simulink model "EISGov_SelectParameter"  (R2016b)
settings: configuration reference "CodeGenConfigSet" (kept outside this file)
values from neighbouring files (symbols this model uses):
  EISGov_SetPLoRmpSlopeNeg_C = Calibration.Parameter    [init_EISGov_SelectParameter.m]    (also in init_EISGov_SelectParameter_SIL.m = Simulink.Parameter)
  EISGov_SetPLoRmpSlopePos_C = Calibration.Parameter    [init_EISGov_SelectParameter.m]    (also in init_EISGov_SelectParameter_SIL.m = Simulink.Parameter)
  EISGov_stPrio_CA = Calibration.Parameter    [init_EISGov_SelectParameter.m]    (also in init_EISGov_SelectParameter_SIL.m = Simulink.Parameter)
undefined symbols (not defined in the file or in its folder): EISGov_num_conv, EISGov_SelectParameter_DT, Switch_conv
libraries: simulink x20, CXLib x3
(part 2 of 2)

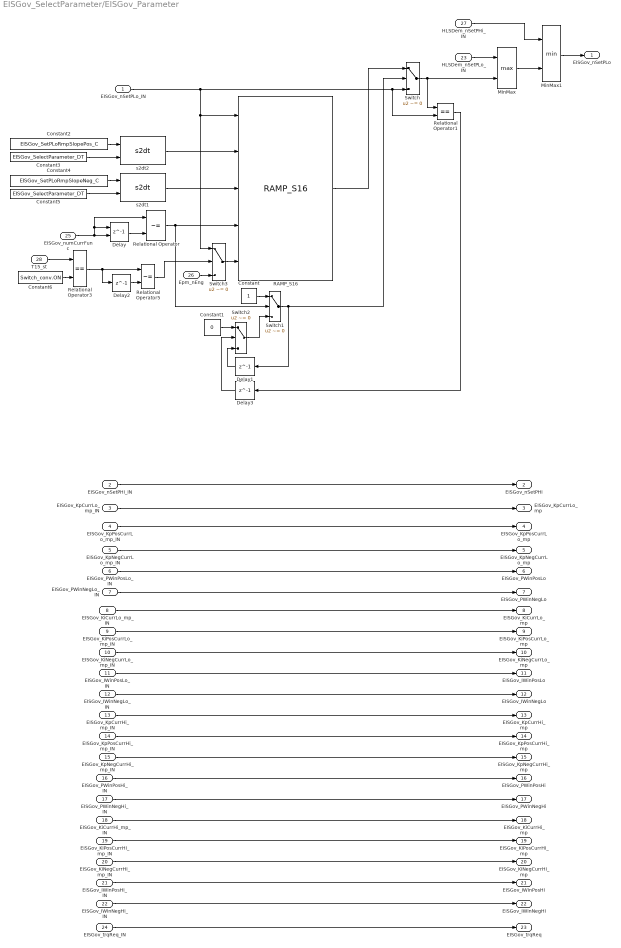
== system EISGov_SelectParameter/EISGov_Parameter ==
  EISGov_nSetPLo_IN : Inport
  EISGov_nSetPHi_IN : Inport  Port=2
  EISGov_KpCurrLo_mp_IN : Inport  Port=3
  EISGov_KpPosCurrLo_mp_IN : Inport  Port=4
  EISGov_KpNegCurrLo_mp_IN : Inport  Port=5
  EISGov_PWinPosLo_IN : Inport  Port=6
  EISGov_PWinNegLo_IN : Inport  Port=7
  EISGov_KiCurrLo_mp_IN : Inport  Port=8
  EISGov_KiPosCurrLo_mp_IN : Inport  Port=9
  EISGov_KiNegCurrLo_mp_IN : Inport  Port=10
  EISGov_IWinPosLo_IN : Inport  Port=11
  EISGov_IWinNegLo_IN : Inport  Port=12
  EISGov_KpCurrHi_mp_IN : Inport  Port=13
  EISGov_KpPosCurrHi_mp_IN : Inport  Port=14
  EISGov_KpNegCurrHi_mp_IN : Inport  Port=15
  EISGov_PWinPosHi_IN : Inport  Port=16
  EISGov_PWinNegHi_IN : Inport  Port=17
  EISGov_KiCurrHi_mp_IN : Inport  Port=18
  EISGov_KiPosCurrHi_mp_IN : Inport  Port=19
  EISGov_KiNegCurrHi_mp_IN : Inport  Port=20
  EISGov_IWinPosHi_IN : Inport  Port=21
  EISGov_IWinNegHi_IN : Inport  Port=22
  HLSDem_nSetPLo_IN : Inport  Port=23
  EISGov_trqReq_IN : Inport  Port=24
  EISGov_numCurrFunc : Inport  Port=25
  Epm_nEng : Inport  Tag=rpm  Description=Engine speed  Port=26  OutMin=0  OutMax=6000  OutDataTypeStr=EngSpeed_rpm
  HLSDem_nSetPHi_IN : Inport  Port=27
  T15_st : Inport  Port=28
  Constant : Constant  OutDataTypeStr=boolean
  Constant1 : Constant  Value=0  OutDataTypeStr=Inherit: Inherit via back propagation
  Constant2 : Constant  Value=EISGov_SetPLoRmpSlopePos_C
  Constant3 : Constant  Value=EISGov_SelectParameter_DT
  Constant4 : Constant  Value=EISGov_SetPLoRmpSlopeNeg_C
  Constant5 : Constant  Value=EISGov_SelectParameter_DT
  Constant6 : Constant  Value=Switch_conv.ON
  Delay : Delay  DelayLength=1  InitialConditionSource=Input port  InitialCondition=0
      settings: InputPortMap=u0,p4
  Delay1 : Delay  DelayLength=1  InitialCondition=0
  Delay2 : Delay  DelayLength=1  InitialCondition=0
  Delay3 : Delay  DelayLength=1  InitialCondition=0
  MinMax : MinMax  Function=max  Inputs=2
  MinMax1 : MinMax  Inputs=2
  RAMP_S16 : CXLib/RAMP_S16
  Relational Operator : RelationalOperator  Operator=~=  OutDataTypeStr=boolean  RndMeth=Simplest
  Relational Operator1 : RelationalOperator  Operator===  OutDataTypeStr=boolean  RndMeth=Simplest
  Relational Operator3 : RelationalOperator  Operator===  OutDataTypeStr=boolean  RndMeth=Simplest
  Relational Operator5 : RelationalOperator  Operator=~=  OutDataTypeStr=boolean  RndMeth=Simplest
  Switch{,1..3} (4 alike) : Switch  Criteria=u2 ~= 0
  s2dt1 : CXLib/s2dt
  s2dt2 : CXLib/s2dt
  EISGov_nSetPLo : Outport
  EISGov_nSetPHi : Outport  Port=2
  EISGov_KpCurrLo_mp : Outport  Port=3
  EISGov_KpPosCurrLo_mp : Outport  Port=4
  EISGov_KpNegCurrLo_mp : Outport  Port=5
  EISGov_PWinPosLo : Outport  Port=6
  EISGov_PWinNegLo : Outport  Port=7
  EISGov_KiCurrLo_mp : Outport  Port=8
  EISGov_KiPosCurrLo_mp : Outport  Port=9
  EISGov_KiNegCurrLo_mp : Outport  Port=10
  EISGov_IWinPosLo : Outport  Port=11
  EISGov_IWinNegLo : Outport  Port=12
  EISGov_KpCurrHi_mp : Outport  Port=13
  EISGov_KpPosCurrHi_mp : Outport  Port=14
  EISGov_KpNegCurrHi_mp : Outport  Port=15
  EISGov_PWinPosHi : Outport  Port=16
  EISGov_PWinNegHi : Outport  Port=17
  EISGov_KiCurrHi_mp : Outport  Port=18
  EISGov_KiPosCurrHi_mp : Outport  Port=19
  EISGov_KiNegCurrHi_mp : Outport  Port=20
  EISGov_IWinPosHi : Outport  Port=21
  EISGov_IWinNegHi : Outport  Port=22
  EISGov_trqReq : Outport  Port=23
  wires:
  EISGov_KpCurrLo_mp_IN/1 -> EISGov_KpCurrLo_mp/1
  EISGov_KpPosCurrLo_mp_IN/1 -> EISGov_KpPosCurrLo_mp/1
  EISGov_nSetPHi_IN/1 -> EISGov_nSetPHi/1
  EISGov_KiCurrLo_mp_IN/1 -> EISGov_KiCurrLo_mp/1
  EISGov_KiPosCurrHi_mp_IN/1 -> EISGov_KiPosCurrHi_mp/1
  EISGov_IWinNegLo_IN/1 -> EISGov_IWinNegLo/1
  EISGov_KpNegCurrHi_mp_IN/1 -> EISGov_KpNegCurrHi_mp/1
  EISGov_KiNegCurrHi_mp_IN/1 -> EISGov_KiNegCurrHi_mp/1
  EISGov_IWinPosLo_IN/1 -> EISGov_IWinPosLo/1
  EISGov_PWinPosHi_IN/1 -> EISGov_PWinPosHi/1
  EISGov_IWinNegHi_IN/1 -> EISGov_IWinNegHi/1
  EISGov_KiPosCurrLo_mp_IN/1 -> EISGov_KiPosCurrLo_mp/1
  EISGov_IWinPosHi_IN/1 -> EISGov_IWinPosHi/1
  EISGov_PWinNegHi_IN/1 -> EISGov_PWinNegHi/1
  EISGov_PWinPosLo_IN/1 -> EISGov_PWinPosLo/1
  EISGov_KpNegCurrLo_mp_IN/1 -> EISGov_KpNegCurrLo_mp/1
  EISGov_PWinNegLo_IN/1 -> EISGov_PWinNegLo/1
  EISGov_KpCurrHi_mp_IN/1 -> EISGov_KpCurrHi_mp/1
  EISGov_KiNegCurrLo_mp_IN/1 -> EISGov_KiNegCurrLo_mp/1
  EISGov_KpPosCurrHi_mp_IN/1 -> EISGov_KpPosCurrHi_mp/1
  EISGov_KiCurrHi_mp_IN/1 -> EISGov_KiCurrHi_mp/1
  HLSDem_nSetPLo_IN/1 -> MinMax/1
  EISGov_trqReq_IN/1 -> EISGov_trqReq/1
  EISGov_numCurrFunc/1 -> Relational Operator/1, Delay/1, Delay/2
  Delay/1 -> Relational Operator/2
  Constant3/1 -> s2dt2/2
  Constant2/1 -> s2dt2/1
  s2dt2/1 -> RAMP_S16/2
  Constant5/1 -> s2dt1/2
  Constant4/1 -> s2dt1/1
  s2dt1/1 -> RAMP_S16/3
  EISGov_nSetPLo_IN/1 -> Relational Operator1/2, Switch/3, RAMP_S16/1, Switch3/1
  Relational Operator/1 -> Switch1/2, RAMP_S16/4
  MinMax1/1 -> EISGov_nSetPLo/1
  MinMax/1 -> MinMax1/2
  HLSDem_nSetPHi_IN/1 -> MinMax1/1
  Switch/1 -> MinMax/2, Relational Operator1/1
  Switch2/1 -> Switch1/3
  Switch1/1 -> Switch/2, Delay1/1
  Constant/1 -> Switch1/1
  Constant1/1 -> Switch2/1
  Delay1/1 -> Switch2/3
  RAMP_S16/1 -> Switch/1
  Constant6/1 -> Relational Operator3/2
  Delay2/1 -> Relational Operator5/2
  Relational Operator3/1 -> Delay2/1, Relational Operator5/1
  T15_st/1 -> Relational Operator3/1
  Epm_nEng/1 -> Switch3/3
  Switch3/1 -> RAMP_S16/5
  Relational Operator5/1 -> Switch3/2
  Delay3/1 -> Switch2/2
  Relational Operator1/1 -> Delay3/1

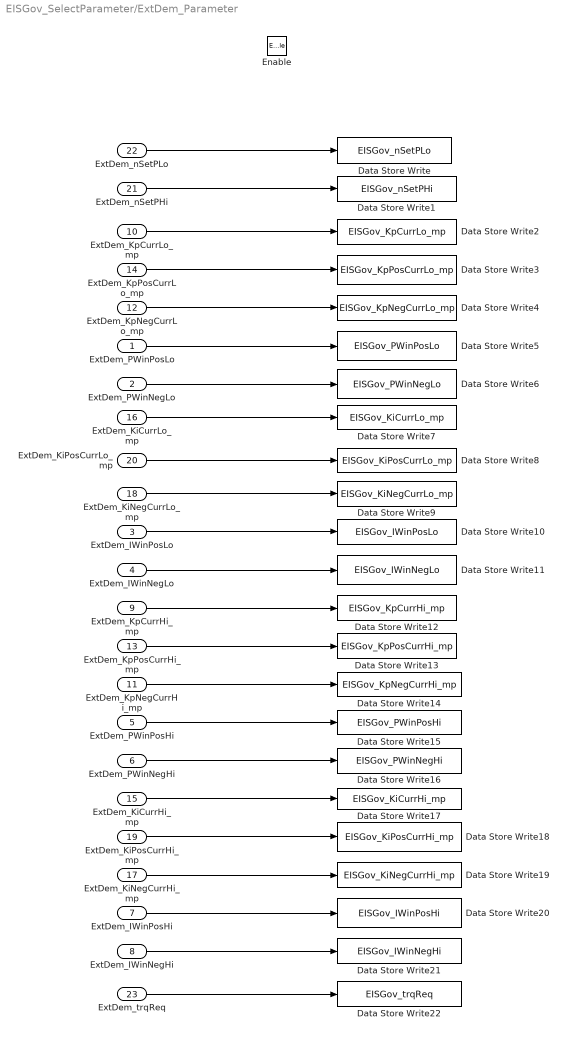
== system EISGov_SelectParameter/ExtDem_Parameter ==
  ExtDem_PWinPosLo : Inport  Tag=rpm  Description=P component Positive window for parameterset lower PI- path  OutMin=-6000  OutMax=6000  OutDataTypeStr=EngSpeed_rpm
  ExtDem_PWinNegLo : Inport  Tag=rpm  Description=P component negative window for parameterset lower PI- path  Port=2  OutMin=-6000  OutMax=6000  OutDataTypeStr=EngSpeed_rpm
  ExtDem_IWinPosLo : Inport  Tag=rpm  Description=I component Positive window for parameterset lower PI- path  Port=3  OutMin=-6000  OutMax=6000  OutDataTypeStr=EngSpeed_rpm
  ExtDem_IWinNegLo : Inport  Tag=rpm  Description=I component negative window for parameterset lower PI- path  Port=4  OutMin=-6000  OutMax=6000  OutDataTypeStr=EngSpeed_rpm
  ExtDem_PWinPosHi : Inport  Tag=rpm  Description=P component Positive window for parameterset upper PI- path  Port=5  OutMin=-6000  OutMax=6000  OutDataTypeStr=EngSpeed_rpm
  ExtDem_PWinNegHi : Inport  Tag=rpm  Description=P component negative window for parameterset upper PI- path  Port=6  OutMin=-6000  OutMax=6000  OutDataTypeStr=EngSpeed_rpm
  ExtDem_IWinPosHi : Inport  Tag=rpm  Description=I component Positive window for parameterset upper PI- path  Port=7  OutMin=-6000  OutMax=6000  OutDataTypeStr=EngSpeed_rpm
  ExtDem_IWinNegHi : Inport  Tag=rpm  Description=I component negative window for parameterset upper PI- path  Port=8  OutMin=-6000  OutMax=6000  OutDataTypeStr=EngSpeed_rpm
  ExtDem_KpCurrHi_mp : Inport  Port=9
  ExtDem_KpCurrLo_mp : Inport  Port=10
  ExtDem_KpNegCurrHi_mp : Inport  Port=11
  ExtDem_KpNegCurrLo_mp : Inport  Port=12
  ExtDem_KpPosCurrHi_mp : Inport  Port=13
  ExtDem_KpPosCurrLo_mp : Inport  Port=14
  ExtDem_KiCurrHi_mp : Inport  Port=15
  ExtDem_KiCurrLo_mp : Inport  Port=16
  ExtDem_KiNegCurrHi_mp : Inport  Port=17
  ExtDem_KiNegCurrLo_mp : Inport  Port=18
  ExtDem_KiPosCurrHi_mp : Inport  Port=19
  ExtDem_KiPosCurrLo_mp : Inport  Port=20
  ExtDem_nSetPHi : Inport  Port=21
  ExtDem_nSetPLo : Inport  Port=22
  ExtDem_trqReq : Inport  Port=23
  Enable : EnablePort
  Data Store Write : DataStoreWrite  DataStoreName=EISGov_nSetPLo
  Data Store Write1 : DataStoreWrite  DataStoreName=EISGov_nSetPHi
  Data Store Write10 : DataStoreWrite  DataStoreName=EISGov_IWinPosLo
  Data Store Write11 : DataStoreWrite  DataStoreName=EISGov_IWinNegLo
  Data Store Write12 : DataStoreWrite  DataStoreName=EISGov_KpCurrHi_mp
  Data Store Write13 : DataStoreWrite  DataStoreName=EISGov_KpPosCurrHi_mp
  Data Store Write14 : DataStoreWrite  DataStoreName=EISGov_KpNegCurrHi_mp
  Data Store Write15 : DataStoreWrite  DataStoreName=EISGov_PWinPosHi
  Data Store Write16 : DataStoreWrite  DataStoreName=EISGov_PWinNegHi
  Data Store Write17 : DataStoreWrite  DataStoreName=EISGov_KiCurrHi_mp
  Data Store Write18 : DataStoreWrite  DataStoreName=EISGov_KiPosCurrHi_mp
  Data Store Write19 : DataStoreWrite  DataStoreName=EISGov_KiNegCurrHi_mp
  Data Store Write2 : DataStoreWrite  DataStoreName=EISGov_KpCurrLo_mp
  Data Store Write20 : DataStoreWrite  DataStoreName=EISGov_IWinPosHi
  Data Store Write21 : DataStoreWrite  DataStoreName=EISGov_IWinNegHi
  Data Store Write22 : DataStoreWrite  DataStoreName=EISGov_trqReq
  Data Store Write3 : DataStoreWrite  DataStoreName=EISGov_KpPosCurrLo_mp
  Data Store Write4 : DataStoreWrite  DataStoreName=EISGov_KpNegCurrLo_mp
  Data Store Write5 : DataStoreWrite  DataStoreName=EISGov_PWinPosLo
  Data Store Write6 : DataStoreWrite  DataStoreName=EISGov_PWinNegLo
  Data Store Write7 : DataStoreWrite  DataStoreName=EISGov_KiCurrLo_mp
  Data Store Write8 : DataStoreWrite  DataStoreName=EISGov_KiPosCurrLo_mp
  Data Store Write9 : DataStoreWrite  DataStoreName=EISGov_KiNegCurrLo_mp
  wires:
  ExtDem_PWinPosLo/1 -> Data Store Write5/1
  ExtDem_PWinNegLo/1 -> Data Store Write6/1
  ExtDem_KiCurrLo_mp/1 -> Data Store Write7/1
  ExtDem_KiPosCurrLo_mp/1 -> Data Store Write8/1
  ExtDem_KiNegCurrLo_mp/1 -> Data Store Write9/1
  ExtDem_IWinPosLo/1 -> Data Store Write10/1
  ExtDem_IWinNegLo/1 -> Data Store Write11/1
  ExtDem_KpCurrHi_mp/1 -> Data Store Write12/1
  ExtDem_KpPosCurrHi_mp/1 -> Data Store Write13/1
  ExtDem_KpNegCurrHi_mp/1 -> Data Store Write14/1
  ExtDem_PWinPosHi/1 -> Data Store Write15/1
  ExtDem_PWinNegHi/1 -> Data Store Write16/1
  ExtDem_KiCurrHi_mp/1 -> Data Store Write17/1
  ExtDem_KiPosCurrHi_mp/1 -> Data Store Write18/1
  ExtDem_KiNegCurrHi_mp/1 -> Data Store Write19/1
  ExtDem_IWinPosHi/1 -> Data Store Write20/1
  ExtDem_IWinNegHi/1 -> Data Store Write21/1
  ExtDem_nSetPLo/1 -> Data Store Write/1
  ExtDem_nSetPHi/1 -> Data Store Write1/1
  ExtDem_KpCurrLo_mp/1 -> Data Store Write2/1
  ExtDem_KpPosCurrLo_mp/1 -> Data Store Write3/1
  ExtDem_KpNegCurrLo_mp/1 -> Data Store Write4/1
  ExtDem_trqReq/1 -> Data Store Write22/1

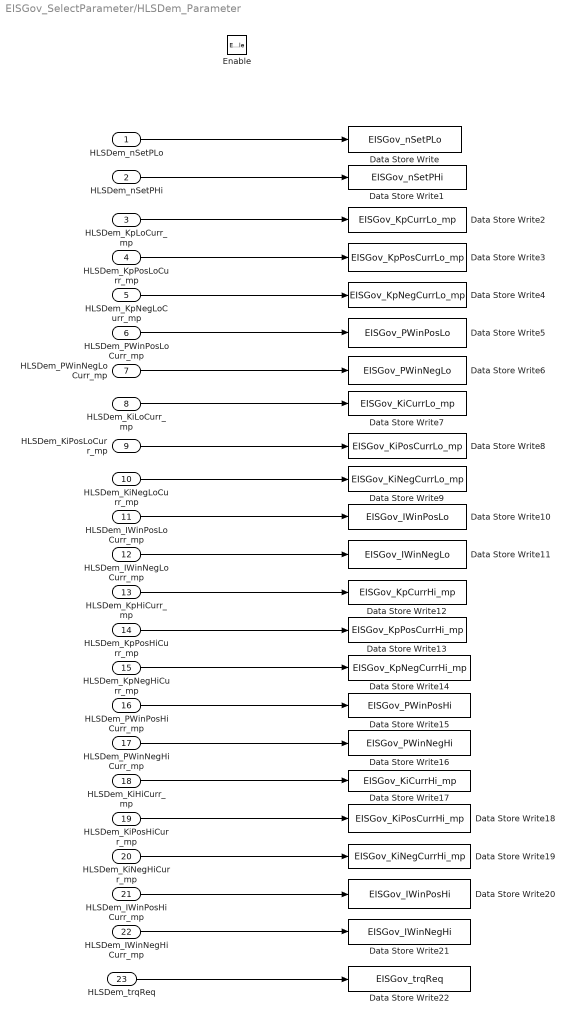
== system EISGov_SelectParameter/HLSDem_Parameter ==
  HLSDem_nSetPLo : Inport
  HLSDem_nSetPHi : Inport  Port=2
  HLSDem_KpLoCurr_mp : Inport  Port=3
  HLSDem_KpPosLoCurr_mp : Inport  Port=4
  HLSDem_KpNegLoCurr_mp : Inport  Port=5
  HLSDem_PWinPosLoCurr_mp : Inport  Port=6
  HLSDem_PWinNegLoCurr_mp : Inport  Port=7
  HLSDem_KiLoCurr_mp : Inport  Port=8
  HLSDem_KiPosLoCurr_mp : Inport  Port=9
  HLSDem_KiNegLoCurr_mp : Inport  Port=10
  HLSDem_IWinPosLoCurr_mp : Inport  Port=11
  HLSDem_IWinNegLoCurr_mp : Inport  Port=12
  HLSDem_KpHiCurr_mp : Inport  Port=13
  HLSDem_KpPosHiCurr_mp : Inport  Port=14
  HLSDem_KpNegHiCurr_mp : Inport  Port=15
  HLSDem_PWinPosHiCurr_mp : Inport  Port=16
  HLSDem_PWinNegHiCurr_mp : Inport  Port=17
  HLSDem_KiHiCurr_mp : Inport  Port=18
  HLSDem_KiPosHiCurr_mp : Inport  Port=19
  HLSDem_KiNegHiCurr_mp : Inport  Port=20
  HLSDem_IWinPosHiCurr_mp : Inport  Port=21
  HLSDem_IWinNegHiCurr_mp : Inport  Port=22
  HLSDem_trqReq : Inport  Port=23
  Enable : EnablePort
  Data Store Write : DataStoreWrite  DataStoreName=EISGov_nSetPLo
  Data Store Write1 : DataStoreWrite  DataStoreName=EISGov_nSetPHi
  Data Store Write10 : DataStoreWrite  DataStoreName=EISGov_IWinPosLo
  Data Store Write11 : DataStoreWrite  DataStoreName=EISGov_IWinNegLo
  Data Store Write12 : DataStoreWrite  DataStoreName=EISGov_KpCurrHi_mp
  Data Store Write13 : DataStoreWrite  DataStoreName=EISGov_KpPosCurrHi_mp
  Data Store Write14 : DataStoreWrite  DataStoreName=EISGov_KpNegCurrHi_mp
  Data Store Write15 : DataStoreWrite  DataStoreName=EISGov_PWinPosHi
  Data Store Write16 : DataStoreWrite  DataStoreName=EISGov_PWinNegHi
  Data Store Write17 : DataStoreWrite  DataStoreName=EISGov_KiCurrHi_mp
  Data Store Write18 : DataStoreWrite  DataStoreName=EISGov_KiPosCurrHi_mp
  Data Store Write19 : DataStoreWrite  DataStoreName=EISGov_KiNegCurrHi_mp
  Data Store Write2 : DataStoreWrite  DataStoreName=EISGov_KpCurrLo_mp
  Data Store Write20 : DataStoreWrite  DataStoreName=EISGov_IWinPosHi
  Data Store Write21 : DataStoreWrite  DataStoreName=EISGov_IWinNegHi
  Data Store Write22 : DataStoreWrite  DataStoreName=EISGov_trqReq
  Data Store Write3 : DataStoreWrite  DataStoreName=EISGov_KpPosCurrLo_mp
  Data Store Write4 : DataStoreWrite  DataStoreName=EISGov_KpNegCurrLo_mp
  Data Store Write5 : DataStoreWrite  DataStoreName=EISGov_PWinPosLo
  Data Store Write6 : DataStoreWrite  DataStoreName=EISGov_PWinNegLo
  Data Store Write7 : DataStoreWrite  DataStoreName=EISGov_KiCurrLo_mp
  Data Store Write8 : DataStoreWrite  DataStoreName=EISGov_KiPosCurrLo_mp
  Data Store Write9 : DataStoreWrite  DataStoreName=EISGov_KiNegCurrLo_mp
  wires:
  HLSDem_nSetPLo/1 -> Data Store Write/1
  HLSDem_nSetPHi/1 -> Data Store Write1/1
  HLSDem_KpLoCurr_mp/1 -> Data Store Write2/1
  HLSDem_KpPosLoCurr_mp/1 -> Data Store Write3/1
  HLSDem_KpNegLoCurr_mp/1 -> Data Store Write4/1
  HLSDem_PWinPosLoCurr_mp/1 -> Data Store Write5/1
  HLSDem_PWinNegLoCurr_mp/1 -> Data Store Write6/1
  HLSDem_KiLoCurr_mp/1 -> Data Store Write7/1
  HLSDem_KiPosLoCurr_mp/1 -> Data Store Write8/1
  HLSDem_KiNegLoCurr_mp/1 -> Data Store Write9/1
  HLSDem_IWinPosLoCurr_mp/1 -> Data Store Write10/1
  HLSDem_IWinNegLoCurr_mp/1 -> Data Store Write11/1
  HLSDem_KpHiCurr_mp/1 -> Data Store Write12/1
  HLSDem_KpPosHiCurr_mp/1 -> Data Store Write13/1
  HLSDem_KpNegHiCurr_mp/1 -> Data Store Write14/1
  HLSDem_PWinPosHiCurr_mp/1 -> Data Store Write15/1
  HLSDem_PWinNegHiCurr_mp/1 -> Data Store Write16/1
  HLSDem_KiHiCurr_mp/1 -> Data Store Write17/1
  HLSDem_KiPosHiCurr_mp/1 -> Data Store Write18/1
  HLSDem_KiNegHiCurr_mp/1 -> Data Store Write19/1
  HLSDem_IWinPosHiCurr_mp/1 -> Data Store Write20/1
  HLSDem_IWinNegHiCurr_mp/1 -> Data Store Write21/1
  HLSDem_trqReq/1 -> Data Store Write22/1

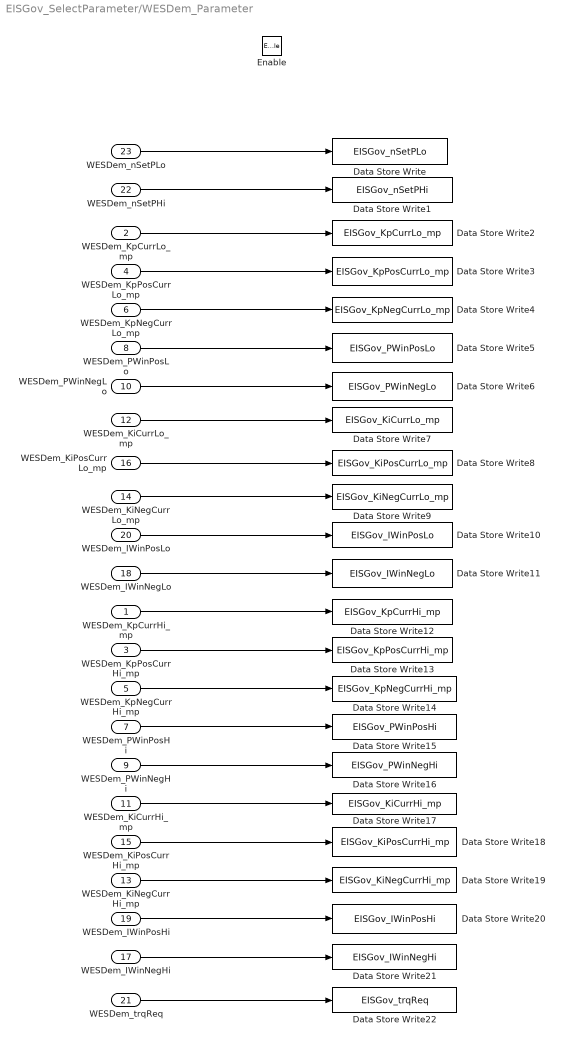
== system EISGov_SelectParameter/WESDem_Parameter ==
  WESDem_KpCurrHi_mp : Inport
  WESDem_KpCurrLo_mp : Inport  Port=2
  WESDem_KpPosCurrHi_mp : Inport  Port=3
  WESDem_KpPosCurrLo_mp : Inport  Port=4
  WESDem_KpNegCurrHi_mp : Inport  Port=5
  WESDem_KpNegCurrLo_mp : Inport  Port=6
  WESDem_PWinPosHi : Inport  Port=7
  WESDem_PWinPosLo : Inport  Port=8
  WESDem_PWinNegHi : Inport  Port=9
  WESDem_PWinNegLo : Inport  Port=10
  WESDem_KiCurrHi_mp : Inport  Port=11
  WESDem_KiCurrLo_mp : Inport  Port=12
  WESDem_KiNegCurrHi_mp : Inport  Port=13
  WESDem_KiNegCurrLo_mp : Inport  Port=14
  WESDem_KiPosCurrHi_mp : Inport  Port=15
  WESDem_KiPosCurrLo_mp : Inport  Port=16
  WESDem_IWinNegHi : Inport  Port=17
  WESDem_IWinNegLo : Inport  Port=18
  WESDem_IWinPosHi : Inport  Port=19
  WESDem_IWinPosLo : Inport  Port=20
  WESDem_trqReq : Inport  Port=21
  WESDem_nSetPHi : Inport  Port=22
  WESDem_nSetPLo : Inport  Port=23
  Enable : EnablePort
  Data Store Write : DataStoreWrite  DataStoreName=EISGov_nSetPLo
  Data Store Write1 : DataStoreWrite  DataStoreName=EISGov_nSetPHi
  Data Store Write10 : DataStoreWrite  DataStoreName=EISGov_IWinPosLo
  Data Store Write11 : DataStoreWrite  DataStoreName=EISGov_IWinNegLo
  Data Store Write12 : DataStoreWrite  DataStoreName=EISGov_KpCurrHi_mp
  Data Store Write13 : DataStoreWrite  DataStoreName=EISGov_KpPosCurrHi_mp
  Data Store Write14 : DataStoreWrite  DataStoreName=EISGov_KpNegCurrHi_mp
  Data Store Write15 : DataStoreWrite  DataStoreName=EISGov_PWinPosHi
  Data Store Write16 : DataStoreWrite  DataStoreName=EISGov_PWinNegHi
  Data Store Write17 : DataStoreWrite  DataStoreName=EISGov_KiCurrHi_mp
  Data Store Write18 : DataStoreWrite  DataStoreName=EISGov_KiPosCurrHi_mp
  Data Store Write19 : DataStoreWrite  DataStoreName=EISGov_KiNegCurrHi_mp
  Data Store Write2 : DataStoreWrite  DataStoreName=EISGov_KpCurrLo_mp
  Data Store Write20 : DataStoreWrite  DataStoreName=EISGov_IWinPosHi
  Data Store Write21 : DataStoreWrite  DataStoreName=EISGov_IWinNegHi
  Data Store Write22 : DataStoreWrite  DataStoreName=EISGov_trqReq
  Data Store Write3 : DataStoreWrite  DataStoreName=EISGov_KpPosCurrLo_mp
  Data Store Write4 : DataStoreWrite  DataStoreName=EISGov_KpNegCurrLo_mp
  Data Store Write5 : DataStoreWrite  DataStoreName=EISGov_PWinPosLo
  Data Store Write6 : DataStoreWrite  DataStoreName=EISGov_PWinNegLo
  Data Store Write7 : DataStoreWrite  DataStoreName=EISGov_KiCurrLo_mp
  Data Store Write8 : DataStoreWrite  DataStoreName=EISGov_KiPosCurrLo_mp
  Data Store Write9 : DataStoreWrite  DataStoreName=EISGov_KiNegCurrLo_mp
  wires:
  WESDem_PWinPosLo/1 -> Data Store Write5/1
  WESDem_PWinNegLo/1 -> Data Store Write6/1
  WESDem_KiCurrLo_mp/1 -> Data Store Write7/1
  WESDem_KiPosCurrLo_mp/1 -> Data Store Write8/1
  WESDem_KiNegCurrLo_mp/1 -> Data Store Write9/1
  WESDem_IWinPosLo/1 -> Data Store Write10/1
  WESDem_IWinNegLo/1 -> Data Store Write11/1
  WESDem_KpCurrHi_mp/1 -> Data Store Write12/1
  WESDem_KpPosCurrHi_mp/1 -> Data Store Write13/1
  WESDem_KpNegCurrHi_mp/1 -> Data Store Write14/1
  WESDem_PWinPosHi/1 -> Data Store Write15/1
  WESDem_PWinNegHi/1 -> Data Store Write16/1
  WESDem_KiCurrHi_mp/1 -> Data Store Write17/1
  WESDem_KiPosCurrHi_mp/1 -> Data Store Write18/1
  WESDem_KiNegCurrHi_mp/1 -> Data Store Write19/1
  WESDem_IWinPosHi/1 -> Data Store Write20/1
  WESDem_IWinNegHi/1 -> Data Store Write21/1
  WESDem_nSetPLo/1 -> Data Store Write/1
  WESDem_nSetPHi/1 -> Data Store Write1/1
  WESDem_KpCurrLo_mp/1 -> Data Store Write2/1
  WESDem_KpPosCurrLo_mp/1 -> Data Store Write3/1
  WESDem_KpNegCurrLo_mp/1 -> Data Store Write4/1
  WESDem_trqReq/1 -> Data Store Write22/1

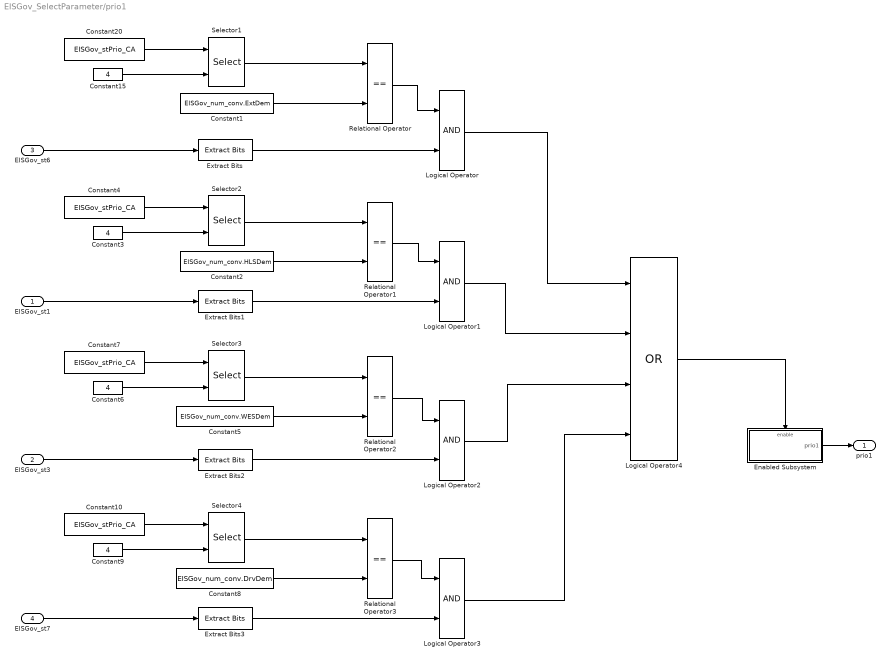
== system EISGov_SelectParameter/prio1 ==
  EISGov_st1 : Inport
  EISGov_st3 : Inport  Port=2
  EISGov_st6 : Inport  Port=3
  EISGov_st7 : Inport  Port=4
  Constant1 : Constant  Value=EISGov_num_conv.ExtDem
  Constant{4,7,10,20} (4 alike) : Constant  Value=EISGov_stPrio_CA
  Constant{3,6,9,15} (4 alike) : Constant  Value=4  OutDataTypeStr=uint8
  Constant2 : Constant  Value=EISGov_num_conv.HLSDem
  Constant5 : Constant  Value=EISGov_num_conv.WESDem
  Constant8 : Constant  Value=EISGov_num_conv.DrvDem
  Enabled Subsystem : Subsystem  TreatAsAtomicUnit=on
  Extract Bits{,1..3} (4 alike) : simulink/Logic and Bit Operations/Extract Bits  bitsToExtract=Range of bits  numBits=8  bitIdxRange=7  outScalingMode=Preserve fixed-point scaling
  Logical Operator{,1..3} (4 alike) : Logic  AllPortsSameDT=off  OutDataTypeStr=boolean
  Logical Operator4 : Logic  Operator=OR  Inputs=4  AllPortsSameDT=off  OutDataTypeStr=boolean
  Relational Operator{,1..3} (4 alike) : RelationalOperator  Operator===  OutDataTypeStr=boolean  RndMeth=Simplest
  Selector{1..4} (4 alike) : Selector  IndexMode=Zero-based  IndexOptions=Index vector (port)  Indices=[1 3]  OutputSizes=1
  prio1 : Outport
  wires:
  Constant20/1 -> Selector1/1
  Constant15/1 -> Selector1/2
  Selector1/1 -> Relational Operator/1
  Logical Operator4/1 -> Enabled Subsystem/Enable
  EISGov_st6/1 -> Extract Bits/1
  Logical Operator/1 -> Logical Operator4/1
  Logical Operator3/1 -> Logical Operator4/4
  Extract Bits/1 -> Logical Operator/2
  Constant10/1 -> Selector4/1
  Constant1/1 -> Relational Operator/2
  Constant8/1 -> Relational Operator3/2
  Relational Operator3/1 -> Logical Operator3/1
  Extract Bits3/1 -> Logical Operator3/2
  EISGov_st7/1 -> Extract Bits3/1
  Selector4/1 -> Relational Operator3/1
  Constant9/1 -> Selector4/2
  Enabled Subsystem/1(prio1) -> prio1/1
  Constant5/1 -> Relational Operator2/2
  Selector3/1 -> Relational Operator2/1
  Constant6/1 -> Selector3/2
  Relational Operator2/1 -> Logical Operator2/1
  Constant7/1 -> Selector3/1
  EISGov_st3/1 -> Extract Bits2/1
  Extract Bits2/1 -> Logical Operator2/2
  Relational Operator/1 -> Logical Operator/1
  Logical Operator1/1 -> Logical Operator4/2
  Extract Bits1/1 -> Logical Operator1/2
  Selector2/1 -> Relational Operator1/1
  Constant4/1 -> Selector2/1
  Constant3/1 -> Selector2/2
  Constant2/1 -> Relational Operator1/2
  EISGov_st1/1 -> Extract Bits1/1
  Relational Operator1/1 -> Logical Operator1/1
  Logical Operator2/1 -> Logical Operator4/3

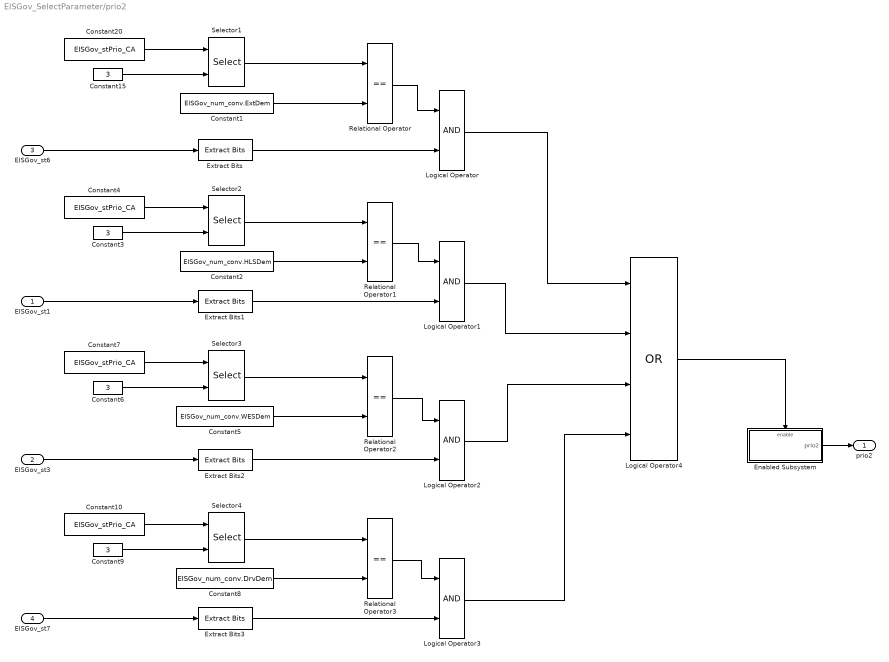
== system EISGov_SelectParameter/prio2 ==
  EISGov_st1 : Inport
  EISGov_st3 : Inport  Port=2
  EISGov_st6 : Inport  Port=3
  EISGov_st7 : Inport  Port=4
  Constant1 : Constant  Value=EISGov_num_conv.ExtDem
  Constant{4,7,10,20} (4 alike) : Constant  Value=EISGov_stPrio_CA
  Constant{3,6,9,15} (4 alike) : Constant  Value=3  OutDataTypeStr=uint8
  Constant2 : Constant  Value=EISGov_num_conv.HLSDem
  Constant5 : Constant  Value=EISGov_num_conv.WESDem
  Constant8 : Constant  Value=EISGov_num_conv.DrvDem
  Enabled Subsystem : Subsystem  TreatAsAtomicUnit=on
  Extract Bits{,1..3} (4 alike) : simulink/Logic and Bit Operations/Extract Bits  bitsToExtract=Range of bits  numBits=8  bitIdxRange=7  outScalingMode=Preserve fixed-point scaling
  Logical Operator{,1..3} (4 alike) : Logic  AllPortsSameDT=off  OutDataTypeStr=boolean
  Logical Operator4 : Logic  Operator=OR  Inputs=4  AllPortsSameDT=off  OutDataTypeStr=boolean
  Relational Operator{,1..3} (4 alike) : RelationalOperator  Operator===  OutDataTypeStr=boolean  RndMeth=Simplest
  Selector{1..4} (4 alike) : Selector  IndexMode=Zero-based  IndexOptions=Index vector (port)  Indices=[1 3]  OutputSizes=1
  prio2 : Outport
  wires:
  Logical Operator2/1 -> Logical Operator4/3
  Relational Operator1/1 -> Logical Operator1/1
  EISGov_st1/1 -> Extract Bits1/1
  Constant2/1 -> Relational Operator1/2
  Constant3/1 -> Selector2/2
  Constant4/1 -> Selector2/1
  Selector2/1 -> Relational Operator1/1
  Extract Bits1/1 -> Logical Operator1/2
  Logical Operator1/1 -> Logical Operator4/2
  Relational Operator/1 -> Logical Operator/1
  Extract Bits2/1 -> Logical Operator2/2
  EISGov_st3/1 -> Extract Bits2/1
  Constant7/1 -> Selector3/1
  Relational Operator2/1 -> Logical Operator2/1
  Constant6/1 -> Selector3/2
  Selector3/1 -> Relational Operator2/1
  Constant5/1 -> Relational Operator2/2
  Enabled Subsystem/1(prio2) -> prio2/1
  Constant9/1 -> Selector4/2
  Selector4/1 -> Relational Operator3/1
  EISGov_st7/1 -> Extract Bits3/1
  Extract Bits3/1 -> Logical Operator3/2
  Relational Operator3/1 -> Logical Operator3/1
  Constant8/1 -> Relational Operator3/2
  Constant1/1 -> Relational Operator/2
  Constant10/1 -> Selector4/1
  Extract Bits/1 -> Logical Operator/2
  Logical Operator3/1 -> Logical Operator4/4
  Logical Operator/1 -> Logical Operator4/1
  EISGov_st6/1 -> Extract Bits/1
  Logical Operator4/1 -> Enabled Subsystem/Enable
  Selector1/1 -> Relational Operator/1
  Constant15/1 -> Selector1/2
  Constant20/1 -> Selector1/1

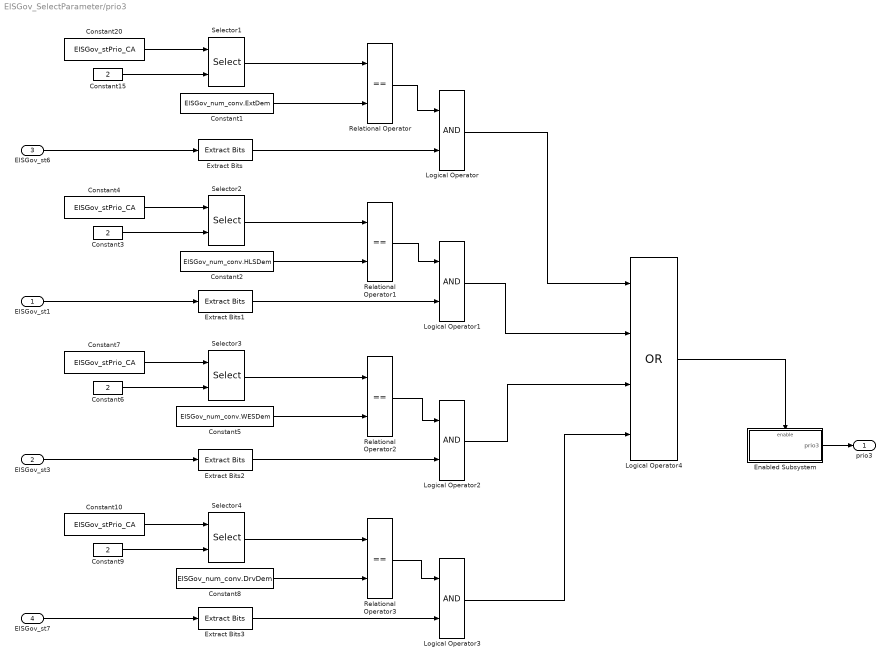
== system EISGov_SelectParameter/prio3 ==
  EISGov_st1 : Inport
  EISGov_st3 : Inport  Port=2
  EISGov_st6 : Inport  Port=3
  EISGov_st7 : Inport  Port=4
  Constant1 : Constant  Value=EISGov_num_conv.ExtDem
  Constant{4,7,10,20} (4 alike) : Constant  Value=EISGov_stPrio_CA
  Constant{3,6,9,15} (4 alike) : Constant  Value=2  OutDataTypeStr=uint8
  Constant2 : Constant  Value=EISGov_num_conv.HLSDem
  Constant5 : Constant  Value=EISGov_num_conv.WESDem
  Constant8 : Constant  Value=EISGov_num_conv.DrvDem
  Enabled Subsystem : Subsystem  TreatAsAtomicUnit=on
  Extract Bits{,1..3} (4 alike) : simulink/Logic and Bit Operations/Extract Bits  bitsToExtract=Range of bits  numBits=8  bitIdxRange=7  outScalingMode=Preserve fixed-point scaling
  Logical Operator{,1..3} (4 alike) : Logic  AllPortsSameDT=off  OutDataTypeStr=boolean
  Logical Operator4 : Logic  Operator=OR  Inputs=4  AllPortsSameDT=off  OutDataTypeStr=boolean
  Relational Operator{,1..3} (4 alike) : RelationalOperator  Operator===  OutDataTypeStr=boolean  RndMeth=Simplest
  Selector{1..4} (4 alike) : Selector  IndexMode=Zero-based  IndexOptions=Index vector (port)  Indices=[1 3]  OutputSizes=1
  prio3 : Outport
  wires:
  Constant20/1 -> Selector1/1
  Constant15/1 -> Selector1/2
  Selector1/1 -> Relational Operator/1
  Logical Operator4/1 -> Enabled Subsystem/Enable
  EISGov_st6/1 -> Extract Bits/1
  Logical Operator/1 -> Logical Operator4/1
  Logical Operator3/1 -> Logical Operator4/4
  Extract Bits/1 -> Logical Operator/2
  Constant10/1 -> Selector4/1
  Constant1/1 -> Relational Operator/2
  Constant8/1 -> Relational Operator3/2
  Relational Operator3/1 -> Logical Operator3/1
  Extract Bits3/1 -> Logical Operator3/2
  EISGov_st7/1 -> Extract Bits3/1
  Selector4/1 -> Relational Operator3/1
  Constant9/1 -> Selector4/2
  Enabled Subsystem/1(prio3) -> prio3/1
  Constant5/1 -> Relational Operator2/2
  Selector3/1 -> Relational Operator2/1
  Constant6/1 -> Selector3/2
  Relational Operator2/1 -> Logical Operator2/1
  Constant7/1 -> Selector3/1
  EISGov_st3/1 -> Extract Bits2/1
  Extract Bits2/1 -> Logical Operator2/2
  Relational Operator/1 -> Logical Operator/1
  Logical Operator1/1 -> Logical Operator4/2
  Extract Bits1/1 -> Logical Operator1/2
  Selector2/1 -> Relational Operator1/1
  Constant4/1 -> Selector2/1
  Constant3/1 -> Selector2/2
  Constant2/1 -> Relational Operator1/2
  EISGov_st1/1 -> Extract Bits1/1
  Relational Operator1/1 -> Logical Operator1/1
  Logical Operator2/1 -> Logical Operator4/3

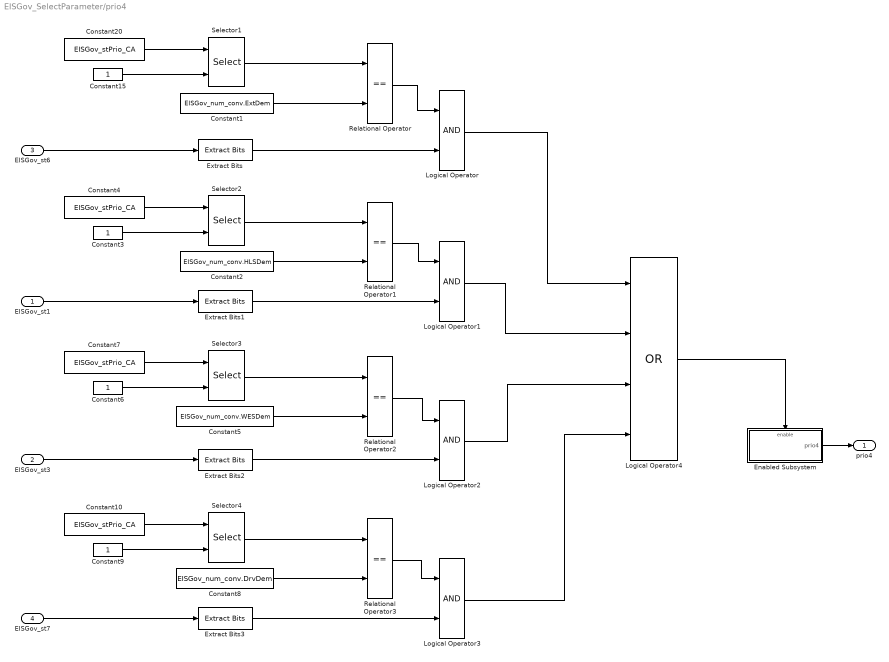
== system EISGov_SelectParameter/prio4 ==
  EISGov_st1 : Inport
  EISGov_st3 : Inport  Port=2
  EISGov_st6 : Inport  Port=3
  EISGov_st7 : Inport  Port=4
  Constant1 : Constant  Value=EISGov_num_conv.ExtDem
  Constant{4,7,10,20} (4 alike) : Constant  Value=EISGov_stPrio_CA
  Constant{3,6,9,15} (4 alike) : Constant  OutDataTypeStr=uint8
  Constant2 : Constant  Value=EISGov_num_conv.HLSDem
  Constant5 : Constant  Value=EISGov_num_conv.WESDem
  Constant8 : Constant  Value=EISGov_num_conv.DrvDem
  Enabled Subsystem : Subsystem  TreatAsAtomicUnit=on
  Extract Bits{,1..3} (4 alike) : simulink/Logic and Bit Operations/Extract Bits  bitsToExtract=Range of bits  numBits=8  bitIdxRange=7  outScalingMode=Preserve fixed-point scaling
  Logical Operator{,1..3} (4 alike) : Logic  AllPortsSameDT=off  OutDataTypeStr=boolean
  Logical Operator4 : Logic  Operator=OR  Inputs=4  AllPortsSameDT=off  OutDataTypeStr=boolean
  Relational Operator{,1..3} (4 alike) : RelationalOperator  Operator===  OutDataTypeStr=boolean  RndMeth=Simplest
  Selector{1..4} (4 alike) : Selector  IndexMode=Zero-based  IndexOptions=Index vector (port)  Indices=[1 3]  OutputSizes=1
  prio4 : Outport
  wires:
  Logical Operator2/1 -> Logical Operator4/3
  Relational Operator1/1 -> Logical Operator1/1
  EISGov_st1/1 -> Extract Bits1/1
  Constant2/1 -> Relational Operator1/2
  Constant3/1 -> Selector2/2
  Constant4/1 -> Selector2/1
  Selector2/1 -> Relational Operator1/1
  Extract Bits1/1 -> Logical Operator1/2
  Logical Operator1/1 -> Logical Operator4/2
  Relational Operator/1 -> Logical Operator/1
  Extract Bits2/1 -> Logical Operator2/2
  EISGov_st3/1 -> Extract Bits2/1
  Constant7/1 -> Selector3/1
  Relational Operator2/1 -> Logical Operator2/1
  Constant6/1 -> Selector3/2
  Selector3/1 -> Relational Operator2/1
  Constant5/1 -> Relational Operator2/2
  Enabled Subsystem/1(prio4) -> prio4/1
  Constant9/1 -> Selector4/2
  Selector4/1 -> Relational Operator3/1
  EISGov_st7/1 -> Extract Bits3/1
  Extract Bits3/1 -> Logical Operator3/2
  Relational Operator3/1 -> Logical Operator3/1
  Constant8/1 -> Relational Operator3/2
  Constant1/1 -> Relational Operator/2
  Constant10/1 -> Selector4/1
  Extract Bits/1 -> Logical Operator/2
  Logical Operator3/1 -> Logical Operator4/4
  Logical Operator/1 -> Logical Operator4/1
  EISGov_st6/1 -> Extract Bits/1
  Logical Operator4/1 -> Enabled Subsystem/Enable
  Selector1/1 -> Relational Operator/1
  Constant15/1 -> Selector1/2
  Constant20/1 -> Selector1/1

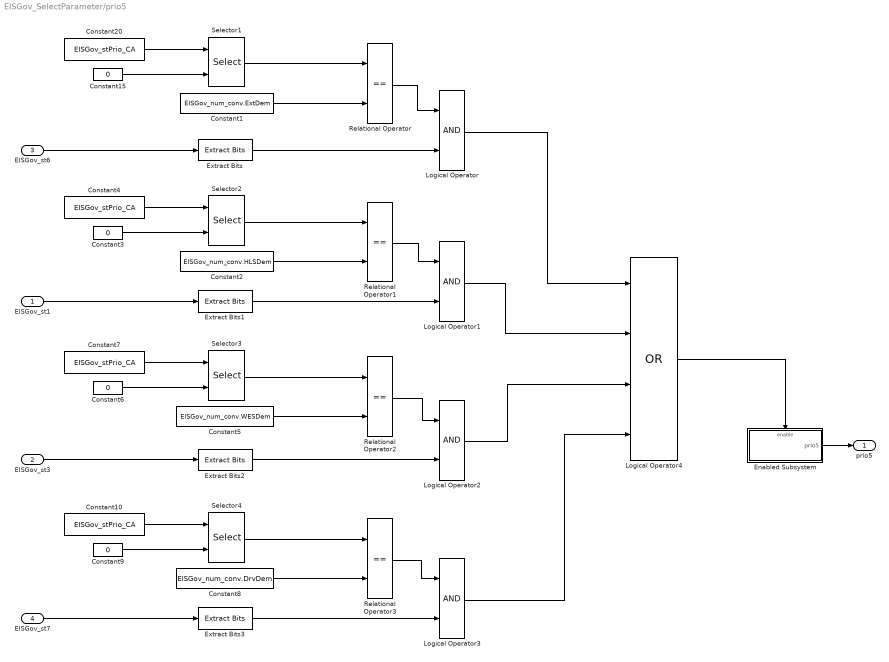
== system EISGov_SelectParameter/prio5 ==
  EISGov_st1 : Inport
  EISGov_st3 : Inport  Port=2
  EISGov_st6 : Inport  Port=3
  EISGov_st7 : Inport  Port=4
  Constant1 : Constant  Value=EISGov_num_conv.ExtDem
  Constant{4,7,10,20} (4 alike) : Constant  Value=EISGov_stPrio_CA
  Constant{3,6,9,15} (4 alike) : Constant  Value=0  OutDataTypeStr=uint8
  Constant2 : Constant  Value=EISGov_num_conv.HLSDem
  Constant5 : Constant  Value=EISGov_num_conv.WESDem
  Constant8 : Constant  Value=EISGov_num_conv.DrvDem
  Enabled Subsystem : Subsystem  TreatAsAtomicUnit=on
  Extract Bits{,1..3} (4 alike) : simulink/Logic and Bit Operations/Extract Bits  bitsToExtract=Range of bits  numBits=8  bitIdxRange=7  outScalingMode=Preserve fixed-point scaling
  Logical Operator{,1..3} (4 alike) : Logic  AllPortsSameDT=off  OutDataTypeStr=boolean
  Logical Operator4 : Logic  Operator=OR  Inputs=4  AllPortsSameDT=off  OutDataTypeStr=boolean
  Relational Operator{,1..3} (4 alike) : RelationalOperator  Operator===  OutDataTypeStr=boolean  RndMeth=Simplest
  Selector{1..4} (4 alike) : Selector  IndexMode=Zero-based  IndexOptions=Index vector (port)  Indices=[1 3]  OutputSizes=1
  prio5 : Outport
  wires:
  Constant20/1 -> Selector1/1
  Constant15/1 -> Selector1/2
  Selector1/1 -> Relational Operator/1
  Logical Operator4/1 -> Enabled Subsystem/Enable
  EISGov_st6/1 -> Extract Bits/1
  Logical Operator/1 -> Logical Operator4/1
  Logical Operator3/1 -> Logical Operator4/4
  Extract Bits/1 -> Logical Operator/2
  Constant10/1 -> Selector4/1
  Constant1/1 -> Relational Operator/2
  Constant8/1 -> Relational Operator3/2
  Relational Operator3/1 -> Logical Operator3/1
  Extract Bits3/1 -> Logical Operator3/2
  EISGov_st7/1 -> Extract Bits3/1
  Selector4/1 -> Relational Operator3/1
  Constant9/1 -> Selector4/2
  Enabled Subsystem/1(prio5) -> prio5/1
  Constant5/1 -> Relational Operator2/2
  Selector3/1 -> Relational Operator2/1
  Constant6/1 -> Selector3/2
  Relational Operator2/1 -> Logical Operator2/1
  Constant7/1 -> Selector3/1
  EISGov_st3/1 -> Extract Bits2/1
  Extract Bits2/1 -> Logical Operator2/2
  Relational Operator/1 -> Logical Operator/1
  Logical Operator1/1 -> Logical Operator4/2
  Extract Bits1/1 -> Logical Operator1/2
  Selector2/1 -> Relational Operator1/1
  Constant4/1 -> Selector2/1
  Constant3/1 -> Selector2/2
  Constant2/1 -> Relational Operator1/2
  EISGov_st1/1 -> Extract Bits1/1
  Relational Operator1/1 -> Logical Operator1/1
  Logical Operator2/1 -> Logical Operator4/3

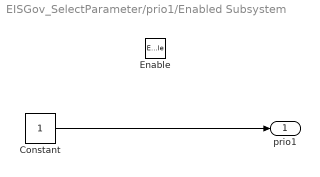
== system EISGov_SelectParameter/prio1/Enabled Subsystem ==
  Enable : EnablePort
  Constant : Constant  OutDataTypeStr=uint8
  prio1 : Outport  OutputWhenDisabled=reset  InitialOutput=0
  wires:
  Constant/1 -> prio1/1

== system EISGov_SelectParameter/prio2/Enabled Subsystem ==
  Enable : EnablePort
  Constant : Constant  Value=2  OutDataTypeStr=uint8
  prio2 : Outport  OutputWhenDisabled=reset  InitialOutput=0
  wires:
  Constant/1 -> prio2/1

== system EISGov_SelectParameter/prio3/Enabled Subsystem ==
  Enable : EnablePort
  Constant : Constant  Value=3  OutDataTypeStr=uint8
  prio3 : Outport  OutputWhenDisabled=reset  InitialOutput=0
  wires:
  Constant/1 -> prio3/1

== system EISGov_SelectParameter/prio4/Enabled Subsystem ==
  Enable : EnablePort
  Constant : Constant  Value=4  OutDataTypeStr=uint8
  prio4 : Outport  OutputWhenDisabled=reset  InitialOutput=0
  wires:
  Constant/1 -> prio4/1

== system EISGov_SelectParameter/prio5/Enabled Subsystem ==
  Enable : EnablePort
  Constant : Constant  Value=5  OutDataTypeStr=uint8
  prio5 : Outport  OutputWhenDisabled=reset  InitialOutput=0
  wires:
  Constant/1 -> prio5/1
